simulink model "lseg2015"  (Simulink 8.6)
settings: Solver=ode45  StartTime=0.0  StopTime=Te  RelTol=1e-3
values from neighbouring files (symbols this model uses):
  A = [0 0 1 0;0 0 0 1;[d1w d2w d3w d4w]]    [fseg.m]
  B = [0 0;0 0;Ui]    [fseg.m]
  C = [1 1 0 0]    [butt.m]    (also in seg.m = [1 0 0 0])
  F = Fl2    [seg.m]
  ue = [0;0]    [seg.m]
undefined symbols (not defined in the file or in its folder): D, ye
libraries: cstblocks x1
settings Model: Creator=cscherer  LastModifiedBy=nemezis
settings OptimizationCC: InitFltsAndDblsToZero=on
settings DebuggingCC: SaveWithParameterizedLinksMsg=none  SignalResolutionControl=TryResolveAllWithWarning  MultiTaskDSMMsg=warning  MultiTaskCondExecSysMsg=none  FcnCallInpInsideContextMsg=EnableAllAsWarning  AllowSymbolicDim=on
settings GRTTargetCC: TargetFcnLib=ansi_tfl_tmw.mat  GeneratePreprocessorConditionals=Use local settings

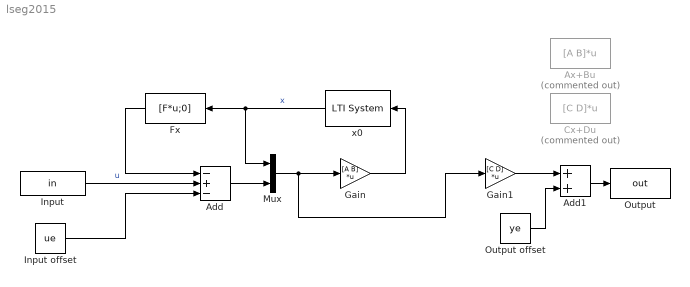
== system lseg2015 ==
  Add : Sum  Inputs=-+-
  Add1 : Sum
  Ax+Bu : MATLABFcn  Commented=on  MATLABFcn=[A B]*u
  Cx+Du : MATLABFcn  Commented=on  MATLABFcn=[C D]*u
  Fx : MATLABFcn  MATLABFcn=[F*u;0]
  Gain : Gain  Gain=[A B]  Multiplication=Matrix(K*u)
  Gain1 : Gain  Gain=[C D]  Multiplication=Matrix(K*u)
  Input : FromWorkspace  VariableName=in  SampleTime=0  OutputAfterFinalValue=Setting to zero
  Input offset : Constant  Value=ue
  Mux : Mux  Inputs=2
  Output : ToWorkspace  VariableName=out  SaveFormat=Structure With Time  SampleTime=-1
  Output offset : Constant  Value=ye
  x0 : cstblocks/LTI System  sys=integrator  IC=x0
  wires:
  Mux/1 -> Gain1/1, Gain/1
  x0/1 -> Mux/1, Fx/1  "x"
  Add/1 -> Mux/2
  Add1/1 -> Output/1
  Output offset/1 -> Add1/2
  Input offset/1 -> Add/3
  Input/1 -> Add/2  "u"
  Fx/1 -> Add/1
  Gain/1 -> x0/1
  Gain1/1 -> Add1/1
